simulink model "cdma"  (R2012b)
settings: Solver=ode45  StartTime=0.0  StopTime=10.0  RelTol=1e-3
undefined symbols (not defined in the file or in its folder): Fs, get, sided, Two
libraries: dspsnks4 x4, commutil2 x2, commsink2 x1, commfilt2 x1, commseqgen2 x1, commrandsrc2 x1, dspsigops x1
settings Model: Creator=mcaceres  LastModifiedBy=mcaceres

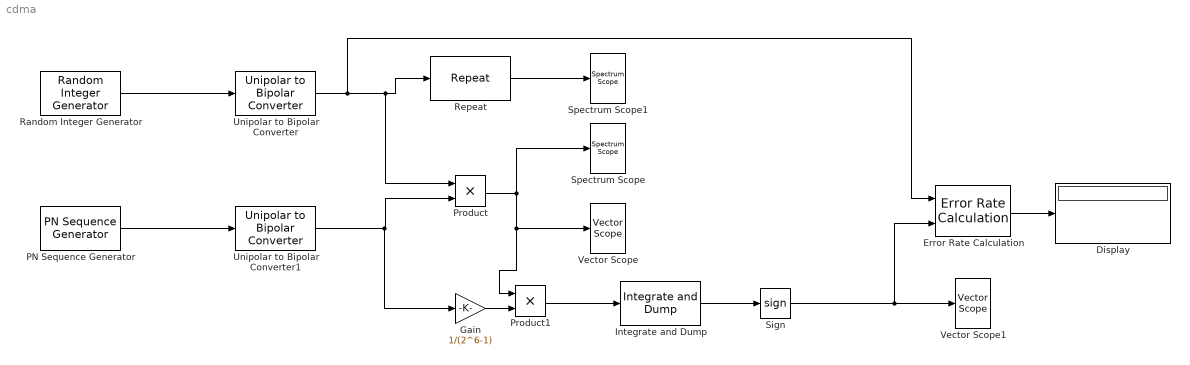
== system cdma ==
  Display : Display
  Error Rate Calculation : commsink2/Error Rate Calculation  N=1  st_delay=0  cp_mode=Entire frame  subframe=[]  PMode=Port  WsName=ErrorVec  RsMode2=off  stop=off  numErr=100  maxBits=1e6
  Gain : Gain  Gain=1/(2^6-1)
  Integrate and Dump : commfilt2/Integrate and Dump  obssamples=63  offsetsamples=0  nodump=off  roundingMode=Floor  overflowMode=off
  PN Sequence Generator : commseqgen2/PN Sequence Generator  poly=[1 1 0 0 0 0 1]  ini_sta=[0 0 0 0 0 1]  outBitMaskSource=Dialog parameter  shift=0  outVarSiz=off  maxOutSizeMode=Dialog parameter  maxOutSize=[10 1]  Ts=(10^-6)/((2^6)-1)  frameBased=off  sampPerFrame=1  reset=off  bitPackedOutputs=off  outDataType=double  numPackedBits=8  bitPackDataSigned=off  bitPackedOutDType=double
  Product : Product  RndMeth=Zero
  Product1 : Product  RndMeth=Zero
  Random Integer Generator : commrandsrc2/Random Integer Generator  mul=2  seed=37  Ts=10^-6  frameBased=off  sampPerFrame=1  orient=off  outDataType=double
  Repeat : dspsigops/Repeat  N=2^6-1  InputProcessing=Columns as channels (frame based)  RateOptions=Allow multirate processing  ic=0  mode=Unused parameter value
  Sign : Signum  ZeroCross=off
  Spectrum Scope : dspsnks4/Spectrum Scope  ScopeProperties=on  Domain=Frequency  HorizSpan=1  UseBuffer=on  BufferSize=128  Overlap=0  TreatMby1Signals=One channel  inpFftLenInherit=on  FFTlength=128  numAvg=20  DisplayProperties=off  AxisGrid=on  Memory=off  FrameNumber=on  AxisLegend=off  AxisZoom=off  OpenScopeAtSimStart=on  OpenScopeImmediately=off  FigPos=get(0,'defaultfigureposition')  AxisProperties=off  XUnits=Hertz  XRange=Two-sided ((-Fs/2...Fs/2])  XDisplay=0  InheritXIncr=on  XIncr=1.0  XLabel=Samples  XLimit=Auto  YUnits=dBW/Hertz  XMax=1  XMin=0  YLabel=Magnitude-squared, dB  LineProperties=off  wintypeSpecScope=Hann  RsSpecScope=50  betaSpecScope=5  winsampSpecScope=Periodic  XAxisParamsVer=6.9  isFrameUpgraded=on
      settings: YMin=-10  YMax=10
  Spectrum Scope1 : dspsnks4/Spectrum Scope  ScopeProperties=on  Domain=Frequency  HorizSpan=1  UseBuffer=on  BufferSize=128  Overlap=0  TreatMby1Signals=One channel  inpFftLenInherit=on  FFTlength=128  numAvg=20  DisplayProperties=off  AxisGrid=on  Memory=off  FrameNumber=on  AxisLegend=off  AxisZoom=off  OpenScopeAtSimStart=on  OpenScopeImmediately=off  FigPos=get(0,'defaultfigureposition')  AxisProperties=off  XUnits=Hertz  XRange=Two-sided ((-Fs/2...Fs/2])  XDisplay=0  InheritXIncr=on  XIncr=1.0  XLabel=Samples  XLimit=Auto  YUnits=dBW/Hertz  XMax=1  XMin=0  YLabel=Magnitude-squared, dB  LineProperties=off  wintypeSpecScope=Hann  RsSpecScope=50  betaSpecScope=5  winsampSpecScope=Periodic  XAxisParamsVer=6.9  isFrameUpgraded=on
      settings: YMin=-10  YMax=10
  Unipolar to Bipolar Converter : commutil2/Unipolar to Bipolar Converter  M=2  polarity=Positive  dataType=Inherit via internal rule
  Unipolar to Bipolar Converter1 : commutil2/Unipolar to Bipolar Converter  M=2  polarity=Positive  dataType=Inherit via internal rule
  Vector Scope : dspsnks4/Vector Scope  ScopeProperties=on  Domain=Time  HorizSpan=3*((2^6)-1)  DisplayProperties=off  AxisGrid=on  Memory=off  FrameNumber=on  AxisLegend=off  AxisZoom=off  OpenScopeAtSimStart=on  OpenScopeImmediately=off  FigPos=get(0,'defaultfigureposition')  AxisProperties=off  XUnits=Hertz  XRange=[0...Fs/2]  InheritXIncr=on  XIncr=1  XLabel=Time  XLimit=Auto  XMin=0  XMax=1  XStart=0  YUnits=dB  YLabel=Amplitude  LineProperties=off  LineStyles=None  LineMarkers=o  XAxisParamsVer=6.9
      settings: YMin=-10  YMax=10
  Vector Scope1 : dspsnks4/Vector Scope  ScopeProperties=on  Domain=Time  HorizSpan=3*((2^6)-1)  DisplayProperties=off  AxisGrid=on  Memory=off  FrameNumber=on  AxisLegend=off  AxisZoom=off  OpenScopeAtSimStart=on  OpenScopeImmediately=off  FigPos=get(0,'defaultfigureposition')  AxisProperties=off  XUnits=Hertz  XRange=[0...Fs/2]  InheritXIncr=on  XIncr=1  XLabel=Time  XLimit=Auto  XMin=0  XMax=1  XStart=0  YUnits=dB  YLabel=Amplitude  LineProperties=off  LineStyles=None  LineMarkers=o  LineColors=b  XAxisParamsVer=6.9
      settings: YMin=-10  YMax=10
  wires:
  Integrate and Dump/1 -> Sign/1
  Error Rate Calculation/1 -> Display/1
  Sign/1 -> Error Rate Calculation/2, Vector Scope1/1
  Gain/1 -> Product1/2
  Product1/1 -> Integrate and Dump/1
  Product/1 -> Product1/1, Vector Scope/1, Spectrum Scope/1
  PN Sequence Generator/1 -> Unipolar to Bipolar Converter1/1
  Unipolar to Bipolar Converter/1 -> Error Rate Calculation/1, Repeat/1, Product/1
  Random Integer Generator/1 -> Unipolar to Bipolar Converter/1
  Repeat/1 -> Spectrum Scope1/1
  Unipolar to Bipolar Converter1/1 -> Gain/1, Product/2
